simulink model "torqueconstantpulses2"  (R2021a)
settings: Solver=VariableStepAuto  StartTime=0.0  StopTime=100  RelTol=1e-3
libraries: spsDiodeLib x4, spsThyristorLib x3, spsACVoltageSourceLib x2, spsGroundLib x2, spsDCMachineLib x1, simulink x1, spspowerguiLib x1
settings Model: Creator=User  LastModifiedBy=User

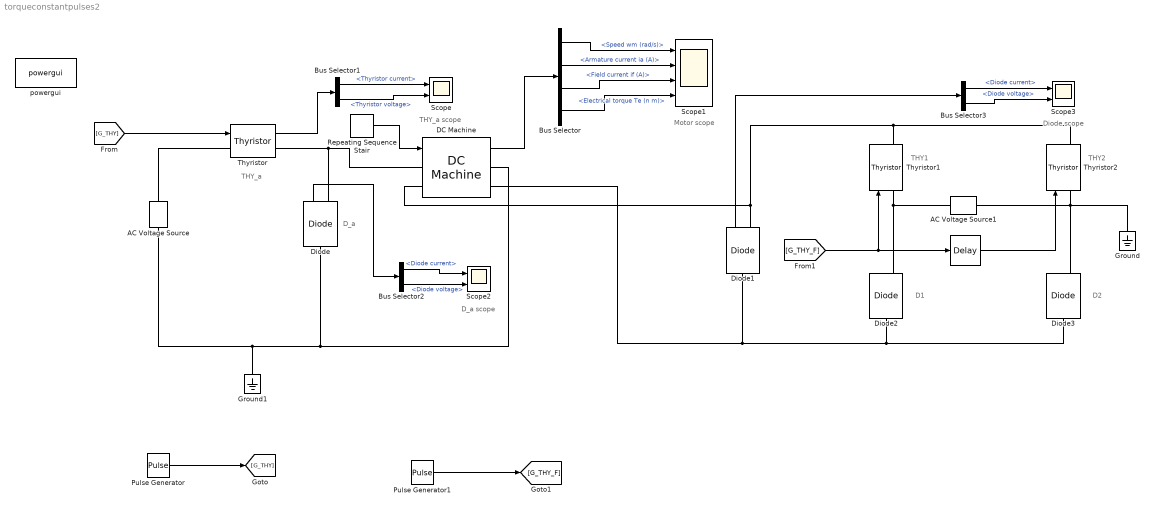
== system torqueconstantpulses2 ==
  note: D_a scope
  note: THY1
  note: D1
  note: THY_a scope
  note: THY2
  note: D_a
  note: Diode scope
  note: Motor scope
  note: THY_a
  note: D2
  " " : TransportDelay  DelayTime=0.01
  AC Voltage Source : spsACVoltageSourceLib/AC Voltage Source  Amplitude=311  Phase=0  Frequency=50  SampleTime=0  Measurements=None  BusType=swing  Pref=10e3  Qref=0  Qmin=-inf  Qmax=+inf
  AC Voltage Source1 : spsACVoltageSourceLib/AC Voltage Source  Amplitude=311  Phase=0  Frequency=50  SampleTime=0  Measurements=None  BusType=swing  Pref=10e3  Qref=0  Qmin=-inf  Qmax=+inf
  Bus Selector : BusSelector  OutputSignals=Speed wm (rad/s),Armature current ia (A),Field current if (A),Electrical torque Te (n m)
  Bus Selector1 : BusSelector  OutputSignals=Thyristor current,Thyristor voltage
  Bus Selector2 : BusSelector  OutputSignals=Diode current,Diode voltage
  Bus Selector3 : BusSelector  OutputSignals=Diode current,Diode voltage
  DC Machine : spsDCMachineLib/DC Machine  PresetModel=04: 10HP 240V 1750RPM Field:300V  MechanicalLoad=Torque TL  FieldType=Wound  ShowDetailedParameters=on  MeasurementBus=off  RLa=[1.086 0.01216]  RLf=[180 71.47]  Laf=0.6458  MachineConstant=Torque constant (N.m/A)  Ke=1.8  Kt=1.8  J=0.04251  Bm=0.003406  Tf=1.046  w0=1  Ifinit=2.13230439421431e-17  TsPowergui=0  TsBlock=-1
  Diode{,1..3} (4 alike) : spsDiodeLib/Diode  Ron=0.001  Lon=0  Vf=0.8  IC=0  UseSnubber=0  Rs=500  Cs=250e-9  Measurements=on
  Ground : spsGroundLib/Ground  LConnTagsString=a
  Ground1 : spsGroundLib/Ground  LConnTagsString=a
  Pulse Generator : DiscretePulseGenerator  PulseType=Time based  Amplitude=10  Period=0.02  PulseWidth=5  PhaseDelay=30*0.02/360
  Pulse Generator1 : DiscretePulseGenerator  PulseType=Time based  Amplitude=10  Period=0.02  PulseWidth=5  PhaseDelay=30*0.02/360
  Repeating Sequence Stair : simulink/Sources/Repeating Sequence Stair  OutValues=[0 0 2 4 -2 ].'  tsamp=6  OutMin=[]  OutMax=[]  OutDataTypeStr=double  OutputDataTypeScalingMode=double  OutDataType=fixdt(0,8)  ConRadixGroup=Best Precision: Vector-wise  OutScaling=2^-12
  Scope : Scope  NumInputPorts=2
  Scope1 : Scope  NumInputPorts=4
  Scope2 : Scope  NumInputPorts=2
  Scope3 : Scope  NumInputPorts=2
  Thyristor : spsThyristorLib/Thyristor  Ron=0.001  Lon=0  Vf=0.8  IC=0  Rs=500  Cs=250e-9  Measurements=on
  Thyristor1 : spsThyristorLib/Thyristor  Ron=0.001  Lon=0  Vf=0.8  IC=0  Rs=500  Cs=250e-9  Measurements=on
  Thyristor2 : spsThyristorLib/Thyristor  Ron=0.001  Lon=0  Vf=0.8  IC=0  Rs=500  Cs=250e-9  Measurements=on
  powergui : spspowerguiLib/powergui  Priority=1  SimulationMode=Continuous  SampleTime=50e-6  frequency=60  Iterations=50  frequencyindice=50  Pbase=100e6  ErrMax=1e-4  UnitsV=kV  UnitsW=MW  buscounter=0  FunctionMessages=off  echomessages=off  EnableUseOfTLC=off  CurrentSourceSwitches=off  DisableSnubberDevices=off  DisableRonSwitches=off  DisableVfSwitches=off  DisplayEquations=off  AutomaticDiscreteSolvers=off  SolverType=Tustin/Backward Euler (TBE)  Interpol=off  ExternalGateDelay=off  methode=off  Ts=100  x0status=blocks  SPID=on  SwTol=0  HookPort=off  NonlinearTolerance=1e-4  nMaxIteration=100  ContinueOnMaxIteration=off  RestoreLinks=warning  ResistiveCurrentMeasurement=off  Frange=[0:2:500]  Ylog=off  Xlog=on  ShowGrid=off  save=off  variable=ZData  structure=0  ZoomFFT=off  StartTime=0.0  cycles=1  DisplayStyle=1  fundamental=60  FreqAxis=off  MaxFrequency=1000  frequencyindicesteady=1  RmsSteady=1  display=off
  wires:
  Repeating Sequence Stair/1 -> DC Machine/1
  Bus Selector3/2 -> Scope3/2  "<Diode voltage>"
  Diode1/1 -> Bus Selector3/1
  Bus Selector1/1 -> Scope/1  "<Thyristor current>"
  Bus Selector1/2 -> Scope/2  "<Thyristor voltage>"
  Diode/1 -> Bus Selector2/1
  " "/1 -> Thyristor2/1
  Bus Selector3/1 -> Scope3/1  "<Diode current>"
  Bus Selector/3 -> Scope1/3  "<Field current if (A)>"
  [G_THY_F] -> Thyristor1/1, " "/1
  Bus Selector/1 -> Scope1/1  "<Speed wm (rad/s)>"
  Bus Selector2/1 -> Scope2/1  "<Diode current>"
  Bus Selector/2 -> Scope1/2  "<Armature current ia (A)>"
  DC Machine/1 -> Bus Selector/1
  [G_THY] -> Thyristor/1
  Bus Selector/4 -> Scope1/4  "<Electrical torque Te (n m)>"
  Thyristor/1 -> Bus Selector1/1
  Bus Selector2/2 -> Scope2/2  "<Diode voltage>"
  Pulse Generator1/1 -> [G_THY_F]
  Pulse Generator/1 -> [G_THY]
  connections:
  DC Machine/RConn1 -- Diode/LConn1 -- Ground1/LConn1 -- AC Voltage Source/LConn1
  Diode3/LConn1 -- Diode1/LConn1 -- DC Machine/RConn2 -- Diode2/LConn1
  Diode2/RConn1 -- AC Voltage Source1/RConn1 -- Thyristor1/LConn1
  Thyristor/RConn1 -- Diode/RConn1 -- DC Machine/LConn1
  Thyristor2/LConn1 -- Ground/LConn1 -- AC Voltage Source1/LConn1 -- Diode3/RConn1
  Diode1/RConn1 -- DC Machine/LConn2 -- Thyristor1/RConn1 -- Thyristor2/RConn1
  AC Voltage Source/RConn1 -- Thyristor/LConn1
